simulink model "receiver_top"  (R2015b)
settings: Solver=VariableStepAuto  StartTime=0.0  StopTime=1  RelTol=1e-3
undefined symbols (not defined in the file or in its folder): magnitude
libraries: dspxfrm3 x3, dspsigops x1, simulink x1
settings Model: Creator=drew  LastModifiedBy=drew

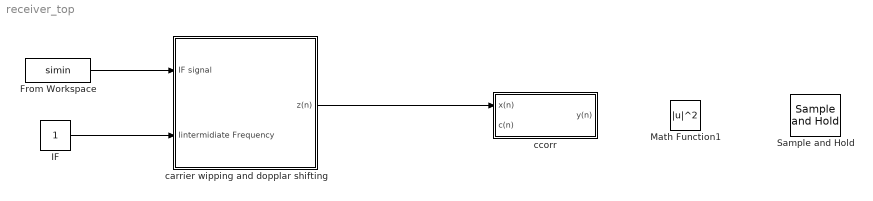
== system receiver_top ==
  From Workspace : FromWorkspace  VariableName=simin  SampleTime=0
  "IF " : Constant
  Math Function1 : Math  Operator=magnitude^2  SaturateOnIntegerOverflow=on
  Sample and Hold : dspsigops/Sample and Hold  trig=Rising edge  initCond=0  latchinput=off
  carrier wipping and dopplar shifting : Subsystem
  ccorr : Subsystem
  wires:
  carrier wipping and dopplar shifting/1(z(n)) -> ccorr/1(x(n))
  From Workspace/1 -> carrier wipping and dopplar shifting/1(IF signal)
  "IF "/1 -> carrier wipping and dopplar shifting/2(Iintermidiate Frequency)

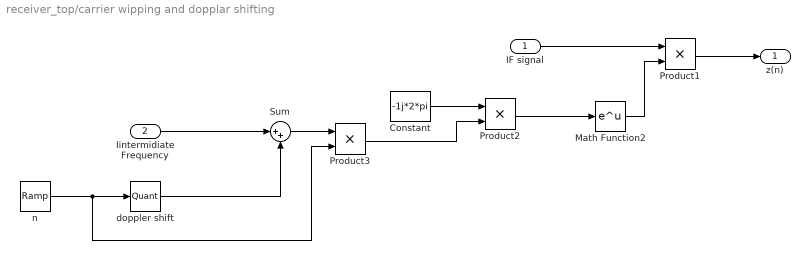
== system receiver_top/carrier wipping and dopplar shifting ==
  IF signal : Inport
  Iintermidiate Frequency : Inport  Port=2
  Constant : Constant  Value=-1j*2*pi
  Math Function2 : Math  OutputSignalType=complex  SaturateOnIntegerOverflow=on
  Product1 : Product
  Product2 : Product
  Product3 : Product
  Sum : Sum  Inputs=|++
  doppler shift : Quantizer
  n : simulink/Sources/Ramp  slope=1  start=0  X0=0
  z(n) : Outport
  wires:
  Math Function2/1 -> Product1/2
  Constant/1 -> Product2/1
  Product2/1 -> Math Function2/1
  IF signal/1 -> Product1/1
  Product1/1 -> z(n)/1
  Product3/1 -> Product2/2
  Sum/1 -> Product3/1
  Iintermidiate Frequency/1 -> Sum/1
  doppler shift/1 -> Sum/2
  n/1 -> Product3/2, doppler shift/1

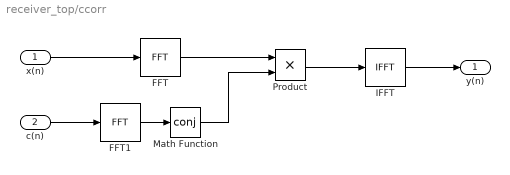
== system receiver_top/ccorr ==
  x(n) : Inport
  c(n) : Inport  Port=2
  FFT : dspxfrm3/FFT  FFTImplementation=Auto  CompMethod=Table lookup  TableOpt=NEW  TableOptActive=Speed  BitRevOrder=off  Normalize=off  InheritFFTLength=on  FFTLength=64  WrapInput=on  roundingMode=Floor  overflowMode=off  firstCoeffDataTypeStr=Inherit: Same word length as input  firstCoeffLastDataTypeStr=Inherit: Same word length as input  outputMin=[]  outputMax=[]
  FFT1 : dspxfrm3/FFT  FFTImplementation=Auto  CompMethod=Table lookup  TableOpt=NEW  TableOptActive=Speed  BitRevOrder=off  Normalize=off  InheritFFTLength=on  FFTLength=64  WrapInput=on  roundingMode=Floor  overflowMode=off  firstCoeffDataTypeStr=Inherit: Same word length as input  firstCoeffLastDataTypeStr=Inherit: Same word length as input  outputMin=[]  outputMax=[]
  IFFT : dspxfrm3/IFFT  FFTImplementation=Auto  CompMethod=Table lookup  TableOpt=NEW  TableOptActive=Speed  BitRevOrder=off  cs_in=off  Normalize=on  InheritFFTLength=on  FFTLength=64  WrapInput=on  mode=Complex  outSamplingMode=Sample based  roundingMode=Floor  overflowMode=off  firstCoeffDataTypeStr=Inherit: Same word length as input  firstCoeffLastDataTypeStr=Inherit: Same word length as input  outputMin=[]  outputMax=[]
  Math Function : Math  Operator=conj  SaturateOnIntegerOverflow=on
  Product : Product
  y(n) : Outport
  wires:
  FFT1/1 -> Math Function/1
  FFT/1 -> Product/1
  Math Function/1 -> Product/2
  Product/1 -> IFFT/1
  x(n)/1 -> FFT/1
  c(n)/1 -> FFT1/1
  IFFT/1 -> y(n)/1
